simulink model "Pendulum_model_nlsysid"  (R2016a)
settings: Solver=ode45  StartTime=0.0  StopTime=10  RelTol=1e-3
values from neighbouring files (symbols this model uses):
  h = 0.01    [generate_step.m]    (also in nonlinid_pendulum.m = diff(time(1:2)))
  k_m = 50    [nonlinid_pendulum.m]
  tau_e = 0.3    [nonlinid_pendulum.m]
  x0 = [pi 0.5*pi 0 0 0]    [nonlinid_pendulum.m]
settings Model: Creator=Nathan  LastModifiedBy=Dick
settings DataIOCC: InitialState=states  LimitDataPoints=on  SaveFormat=Array
settings DebuggingCC: AllowSymbolicDim=off
settings HardwareCC: ProdBitPerPointer=32  ProdLargestAtomicFloat=None  ProdIntDivRoundTo=Undefined  ProdEndianess=Unspecified  ProdWordSize=32  ProdHWDeviceType=32-bit Generic
settings ModelReferenceCC: PropagateSignalLabelsOutOfModel=off
settings ConfigComp: CovModelRefEnable=Off

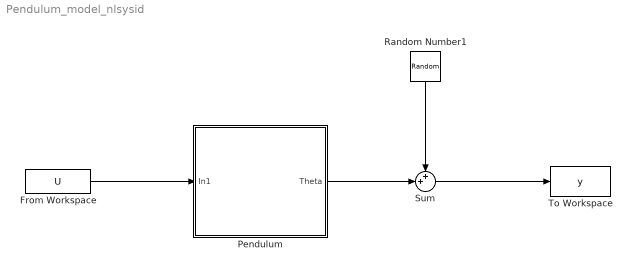
== system Pendulum_model_nlsysid ==
  From Workspace : FromWorkspace  VariableName=U  SampleTime=h
  Pendulum : Subsystem
  Random Number1 : RandomNumber  Variance=1e-4  SampleTime=h
  Sum : Sum  Inputs=++|
  To Workspace : ToWorkspace  VariableName=y  SampleTime=h
  wires:
  Pendulum/1(Theta) -> Sum/2
  Random Number1/1 -> Sum/1
  Sum/1 -> To Workspace/1
  From Workspace/1 -> Pendulum/1(In1)

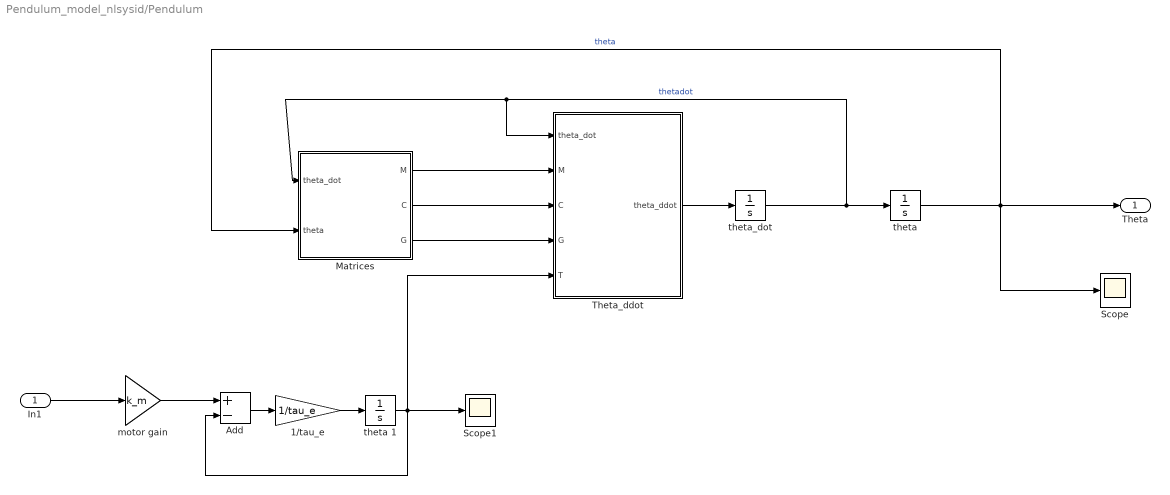
== system Pendulum_model_nlsysid/Pendulum ==
  In1 : Inport
  "1/tau_e " : Gain  Gain=1/tau_e
  Add : Sum  Inputs=+-
  Matrices : MATLAB Function  TreatAsAtomicUnit=on
  Scope : Scope
  Scope1 : Scope
  "Theta_ddot " : MATLAB Function  TreatAsAtomicUnit=on
  "motor gain " : Gain  Gain=k_m
  "theta " : Integrator  InitialCondition=[x0(1) x0(2)]
  theta 1 : Integrator  InitialCondition=x0(5)
  "theta_dot " : Integrator  InitialCondition=[x0(3) x0(4)]
  Theta : Outport
  wires:
  theta 1/1 -> "Theta_ddot "/5(T), Scope1/1, Add/2
  "1/tau_e "/1 -> theta 1/1
  Add/1 -> "1/tau_e "/1
  "motor gain "/1 -> Add/1
  "theta "/1 -> Theta/1, Scope/1, Matrices/2(theta)  "theta"
  "theta_dot "/1 -> "theta "/1, "Theta_ddot "/1(theta_dot), Matrices/1(theta_dot)  "thetadot"
  "Theta_ddot "/1(theta_ddot) -> "theta_dot "/1
  Matrices/3(G) -> "Theta_ddot "/4(G)
  Matrices/2(C) -> "Theta_ddot "/3(C)
  Matrices/1(M) -> "Theta_ddot "/2(M)
  In1/1 -> "motor gain "/1

== matlab function Pendulum_model_nlsysid/Pendulum/Theta_ddot  ==
  data: theta_dot input; M input; C input; G input; theta_ddot output; T input
function theta_ddot = fcn(theta_dot,M,C,G,T)
theta_ddot = [0;0];

theta_ddot = M\[T;0] - M\C*theta_dot - M\G;

== matlab function Pendulum_model_nlsysid/Pendulum/Matrices ==
  data: theta_dot input; theta input; M output; C output; G output
function [M, C, G] = fcn(theta_dot, theta)

M = zeros(2);
C = zeros(2);
G = [0;0];

g = 9.81; 
l1 = 0.1;
l2 = 0.1;
m1 = 0.125;
m2 = 0.05;
c1 = -0.04; % Keeping it negative results in no motion at all, -0.04 or + 0.04?
c2 = 0.06;
I1 = 0.074;
I2 = 0.00012;
b1 = 4.8;
b2 = 0.0002;

P1 = m1*c1^2+m2*l1^2+I1;
P2 = m2*c2^2+ I2;
P3 = m2*l1*c2;
g1 = (m1*c1+m2*l1)*g;
g2 = m2*c2*g;

M = [(P1 + P2 + 2*P3*cos(theta(2)))               (P2 + P3*cos(theta(2))) ;
     (P2 + P3*cos(theta(2)))                       P2                   ];
 
 
C = [(b1 - P3*theta_dot(2)*sin(theta(2)))           (-P3*(theta_dot(1)+theta_dot(2))*sin(theta(2))) ;
     (P3*theta_dot(1)*sin(theta(2)))                 b2                                      ];
     
G = [(-g1*sin(theta(1))-g2*sin(theta(1) + theta(2))) ;
      -g2*sin(theta(1)+theta(2))                   ];
